simulink model "lab_6b_model"  (R2013b)
settings: Solver=ode1  StartTime=0.0  StopTime=10  FixedStep=0.002  RelTol=1e-3
values from neighbouring files (symbols this model uses):
  A = [0, 1, 0, 0 ... (first row only)    [Runner.m]    (also in sine_ref_ws.mat = [0 0 0 0 1 -6.81227956989 0 15.4730759462 0 -1.49726820276 0; zero_ref_perturb_ws.mat = [0 0 0 0 1 -6.81227956989 0 15.4730759462 0 -1.49726820276 0; zero_ref_workspace.mat = [0 0 0 0 1 -6.81227956989 0 15.4730759462 0 -1.49726820276 0)
  B = [0; b_2; 0; b_4]    [Runner.m]    (also in sine_ref_ws.mat = [0 1.52258064516 0 -3.45831460894]; zero_ref_perturb_ws.mat = [0 1.52258064516 0 -3.45831460894]; zero_ref_workspace.mat = [0 1.52258064516 0 -3.45831460894])
  C = [1, 0, 0, 0 ... (first row only)    [Runner.m]    (also in sine_ref_ws.mat = [1  0  0  0; 0  0  1  0]; zero_ref_perturb_ws.mat = [1  0  0  0; 0  0  1  0]; zero_ref_workspace.mat = [1  0  0  0; 0  0  1  0])
  K = [-13.0283303673756 -14.7848226904404 -48.1649225128586 -6.6213771417843]    [Runner.m]    (also in sine_ref_ws.mat = [-13.0283303674 -14.7848226904 -48.1649225129 -6.62137714178; zero_ref_perturb_ws.mat = [-13.0283303674 -14.7848226904 -48.1649225129 -6.62137714178; zero_ref_workspace.mat = [-13.0283303674 -14.7848226904 -48.1649225129 -6.62137714178)
  L = [16.1595   -2.3767 ... (first row only)    [Runner.m]    (also in sine_ref_ws.mat = [16.1595  -2.3767; 254.9779  -5.4833; 15.7136  21.0282; 180.; zero_ref_perturb_ws.mat = [16.1595  -2.3767; 254.9779  -5.4833; 15.7136  21.0282; 180.; zero_ref_workspace.mat = [16.1595  -2.3767; 254.9779  -5.4833; 15.7136  21.0282; 180.)
undefined symbols (not defined in the file or in its folder): HIL
libraries: quarc_library x3
settings Model: SimulationMode=external  ExtModeTrigDuration=50000  Creator=ee128-abc  LastModifiedBy=ee128-abc
settings SolverCC: PositivePriorityOrder=on
settings DataIOCC: LimitDataPoints=off
settings RTWCC: SystemTargetFile=quarc_win64.tlc  TemplateMakefile=quarc_default_tmf  Description=QUARC Win64 Target  ProcessScript=quarc_win64_make_rtw_hook
settings STFCustomTargetCC: TargetPreCompLibLocation=C:\PROGRA~3\QUARC\lib\2013b\win64\release  GeneratePreprocessorConditionals=Disable all  CombineOutputUpdateFcns=on  GRTInterface=off  SystemTargetFile=quarc_win64.tlc
settings GRTTargetCC: TargetPreCompLibLocation=C:\PROGRA~3\QUARC\lib\2013b\win64\release  ParMdlRefBuildCompliant=off  CompOptLevelCompliant=off  ConcurrentExecutionCompliant=off  MatFileLogging=off  ExtMode=on  ExtModeMexFile=quarc_comm

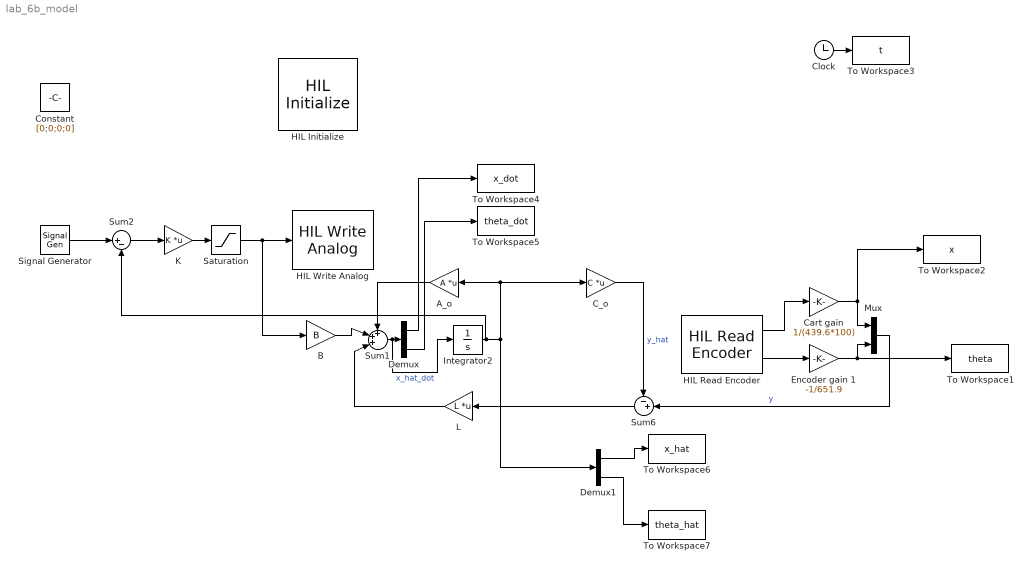
== system lab_6b_model ==
  A_o : Gain  Gain=A  Multiplication=Matrix(K*u)
  B : Gain  Gain=B
  C_o : Gain  Gain=C  Multiplication=Matrix(K*u)
  "Cart gain " : Gain  Gain=1/(439.6*100)
  Clock : Clock
  Constant : Constant  Value=[0;0;0;0]
  Demux : Demux  Outputs=2
  Demux1 : Demux  Outputs=2
  Encoder gain 1 : Gain  Gain=-1/651.9
  HIL Initialize : quarc_library/Data Acquisition/Generic/Configuration/HIL Initialize  Priority=-99  object_name=HIL-1  board_type=q4  board_number=0  exclusive=off  active=off  hardware_clocks=[0:1]  clock_modes=[0 0]  initial_clock_frequencies=[]  set_clock_params_at_start=on  set_clock_params_at_switch_in=off  set_clock_frequencies_at_start=off  set_clock_frequencies_at_switch_in=off  analog_input_channels=[0:3]  analog_input_maximums=10  analog_input_minimums=-10  set_analog_input_params_at_start=off  set_analog_input_params_at_switch_in=off  analog_output_channels=[0:3]  analog_output_maximums=[10]  analog_output_minimums=[-10]  initial_analog_outputs=[0]  final_analog_outputs=[0]  watchdog_analog_outputs=0  set_analog_output_params_at_start=on  set_analog_output_params_at_switch_in=off  set_analog_outputs_at_start=on  set_analog_outputs_at_switch_in=off  set_analog_outputs_at_terminate=on  set_analog_outputs_at_switch_out=off  set_analog_outputs_on_watchdog=off  digital_input_channels=[]  digital_output_channels=[]  digital_output_configuration=[]  initial_digital_outputs=[1]  final_digital_outputs=[1]  watchdog_digital_outputs=[2]  set_digital_output_params_at_start=off  set_digital_output_params_at_switch_in=off  set_digital_outputs_at_start=on  set_digital_outputs_at_switch_in=off  set_digital_outputs_at_terminate=on  set_digital_outputs_at_switch_out=off  set_digital_outputs_on_watchdog=off  encoder_channels=[0:3]  quadrature=[4]  encoder_filter_frequency=(1/60e-9)/1  initial_encoder_counts=[0]  set_encoder_params_at_start=on  set_encoder_params_at_switch_in=off  set_encoder_counts_at_start=on  set_encoder_counts_at_switch_in=off  pwm_channels=[]  pwm_modes=[0]  pwm_frequency=(1/60e-9)/1024  pwm_configuration=[]  pwm_alignment=[]  pwm_polarity=[]  pwm_leading_deadband=[]  pwm_trailing_deadband=[]  initial_pwm_outputs=[0]  final_pwm_outputs=[0]  watchdog_pwm_outputs=[]  set_pwm_params_at_start=on  set_pwm_params_at_switch_in=off  set_pwm_outputs_at_start=on  set_pwm_outputs_at_switch_in=off  set_pwm_outputs_at_terminate=on  set_pwm_outputs_at_switch_out=off  set_pwm_outputs_on_watchdog=off  other_output_channels=[]  initial_other_outputs=[]  final_other_outputs=[]  watchdog_other_outputs=[]  set_other_outputs_at_start=off  set_other_outputs_at_switch_in=off  set_other_outputs_at_terminate=off  set_other_outputs_at_switch_out=off  set_other_outputs_on_watchdog=off
  HIL Read Encoder : quarc_library/Data Acquisition/Generic/Immediate I//O/HIL Read Encoder  object_name=HIL-1  channels=[0, 1]  sample_time=qc_get_step_size  active=on  vector_output=off  data_type_mode=Inherit via back propagation  data_type=double
  HIL Write Analog : quarc_library/Data Acquisition/Generic/Immediate I//O/HIL Write Analog  object_name=HIL-1  channels=0  sample_time=-1  active=off  vector_input=off
  Integrator2 : Integrator  InitialCondition=[0; 0; 0; 0]
  "K " : Gain  Gain=K  Multiplication=Matrix(K*u)
  "L " : Gain  Gain=L  Multiplication=Matrix(K*u)
  Mux : Mux  Inputs=2
  Saturation : Saturate  UpperLimit=6  LowerLimit=-6
  Signal Generator : SignalGenerator  Amplitude=[.05, 0, 0, 0]  Units=rad/sec
  Sum1 : Sum  Inputs=+++|
  Sum2 : Sum  Inputs=|+-
  Sum6 : Sum  Inputs=-+|
  To Workspace1 : ToWorkspace  VariableName=theta  SampleTime=-1
  To Workspace2 : ToWorkspace  VariableName=x  SampleTime=-1
  To Workspace3 : ToWorkspace  VariableName=t  SampleTime=-1
  To Workspace4 : ToWorkspace  VariableName=x_dot  SampleTime=-1
  To Workspace5 : ToWorkspace  VariableName=theta_dot  SampleTime=-1
  To Workspace6 : ToWorkspace  VariableName=x_hat  SampleTime=-1
  To Workspace7 : ToWorkspace  VariableName=theta_hat  SampleTime=-1
  wires:
  Integrator2/1 -> Sum2/2, Demux1/1, C_o/1, A_o/1
  HIL Read Encoder/1 -> "Cart gain "/1
  HIL Read Encoder/2 -> Encoder gain 1/1
  "Cart gain "/1 -> Mux/1, To Workspace2/1
  Encoder gain 1/1 -> To Workspace1/1, Mux/2
  Mux/1 -> Sum6/2  "y"
  Sum6/1 -> "L "/1
  B/1 -> Sum1/2
  "L "/1 -> Sum1/3
  A_o/1 -> Sum1/1
  C_o/1 -> Sum6/1  "y_hat"
  Saturation/1 -> B/1, HIL Write Analog/1
  Sum2/1 -> "K "/1
  "K "/1 -> Saturation/1
  Clock/1 -> To Workspace3/1
  Sum1/1 -> Integrator2/1, Demux/1  "x_hat_dot"
  Demux/1 -> To Workspace4/1
  Demux/2 -> To Workspace5/1
  Demux1/1 -> To Workspace6/1
  Demux1/2 -> To Workspace7/1
  Signal Generator/1 -> Sum2/1
